simulink model "planning"  (R2018b)
settings: Solver=FixedStepDiscrete  StartTime=0.0  StopTime=10.0  RelTol=1e-3
settings Model: ExtModeTrigDuration=2  Creator=sin29  LastModifiedBy=sin29
settings OptimizationCC: DefaultParameterBehavior=Inlined  UseDivisionForNetSlopeComputation=on  UseFloatMulNetSlope=on  InlineInvariantSignals=on  PassReuseOutputArgsAs=Individual arguments  ZeroExternalMemoryAtStartup=off  ZeroInternalMemoryAtStartup=off  NoFixptDivByZeroProtection=on  EfficientFloat2IntCast=on  LifeSpan=1  MaxStackSize=64  OptimizeBlockOrder=speed  DifferentSizesBufferReuse=on
settings DebuggingCC: ParameterTunabilityLossMsg=error
settings HardwareCC: ProdBitPerInt=16  ProdBitPerPointer=16  ProdBitPerSizeT=16  ProdBitPerPtrDiffT=16  ProdLargestAtomicFloat=None  ProdWordSize=8  ProdLongLongMode=on  ProdHWDeviceType=Atmel->AVR
settings SFSimCC: MATLABDynamicMemAlloc=off
settings RTWCC: SystemTargetFile=ert.tlc  HardwareBoard=Arduino Uno  TemplateMakefile=ert_default_tmf  GenerateReport=on  Toolchain=Arduino AVR  BuildConfiguration=Faster Runs  IncludeHyperlinkInReport=on  LaunchReport=on  GenerateTraceInfo=on  GenerateTraceReport=on  GenerateTraceReportSl=on  GenerateTraceReportSf=on  GenerateTraceReportEml=on  GenerateCodeMetricsReport=on
settings CodeAppCC: ForceParamTrailComments=on  IgnoreCustomStorageClasses=off  OperatorAnnotations=on  SimulinkDataObjDesc=on  SFDataObjDesc=on  CustomSymbolStrGlobalVar=rt$N$M  CustomSymbolStrType=$N$M  CustomSymbolStrFcn=$N$M$F  CustomSymbolStrMacro=$N$M  InsertBlockDesc=on
settings ERTTargetCC: IncludeMdlTerminateFcn=off  CombineSignalStateStructs=on  SupportAbsoluteTime=off  SupportComplex=off  SupportNonInlinedSFcns=on  InlinedParameterPlacement=NonHierarchical  ERTFilePackagingFormat=CompactWithDataFile

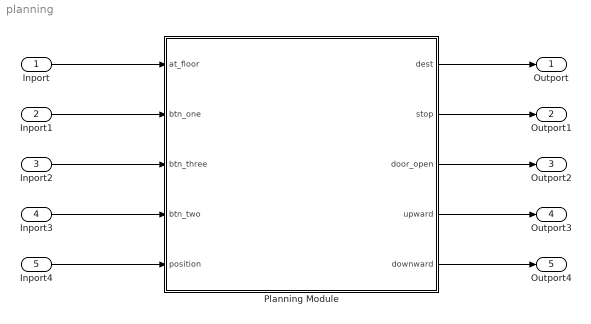
== system planning ==
  Inport : Inport
  Inport1 : Inport  Port=2
  Inport2 : Inport  Port=3
  Inport3 : Inport  Port=4
  Inport4 : Inport  Port=5
  "Planning Module " : Stateflow chart  TreatAsAtomicUnit=on
  Outport : Outport
  Outport1 : Outport  Port=2
  Outport2 : Outport  Port=3
  Outport3 : Outport  Port=4
  Outport4 : Outport  Port=5
  wires:
  Inport/1 -> "Planning Module "/1(at_floor)
  Inport1/1 -> "Planning Module "/2(btn_one)
  Inport2/1 -> "Planning Module "/3(btn_three)
  Inport3/1 -> "Planning Module "/4(btn_two)
  Inport4/1 -> "Planning Module "/5(position)
  "Planning Module "/1(dest) -> Outport/1
  "Planning Module "/2(stop) -> Outport1/1
  "Planning Module "/3(door_open) -> Outport2/1
  "Planning Module "/4(upward) -> Outport3/1
  "Planning Module "/5(downward) -> Outport4/1

== stateflow chart planning/Planning Module  ==
  state planning_cal
    state plan_handle [parallel]
      settings: executionOrder=1
      state floor1
        entry:
        one_pressed = 0;
        door_open = 1;
        stop = 1;
      state floor3
        entry:
        three_pressed = 0;
        door_open = 1;
        stop = 1;
      state move_up
        entry:
        door_open = 0;
        stop = 0;
        upward = 1;
        downward = 0;
      state move_down
        entry:
        door_open = 0;
        stop = 0;
        upward = 0;
        downward = 1;
      state floor2
        entry:
        two_pressed = 0;
        door_open = 1;
        stop = 1;
      floor1 -> floor1 [order 1] : [one_pressed == 1]
      (default) -> floor1
      floor1 -> move_up [order 2] : [after(5, sec) && two_pressed == 1]{dest = 2; two_open = 1}
      move_down -> floor1 [order 3] : [one_pressed == 1 && at_floor == 1]
      floor1 -> move_up [order 3] : [after(5, sec) && two_pressed == 0 && three_pressed == 1]{dest = 3; two_open = 0}
      floor3 -> floor3 [order 1] : [three_pressed == 1]
      move_up -> move_up [order 1] : [two_pressed == 1 && two_open == 0 && position <= 200]{two_open = 1; dest = 2}
      move_up -> floor3 [order 3] : [three_pressed == 1 && at_floor == 3]
      floor3 -> move_down [order 2] : [after(5, sec) && two_pressed == 0 && one_pressed == 1]{dest = 1; two_open = 0}
      floor3 -> move_down [order 3] : [after(5, sec) && two_pressed == 1]{dest = 2; two_open = 1}
      floor2 -> move_up [order 2] : [after(5, sec) && three_pressed == 1]{dest = 3}
      move_up -> floor2 [order 2] : [at_floor == 2 && two_pressed == 1 && two_open == 1]
      floor2 -> floor2 [order 1] : [two_pressed == 1]
      move_down -> floor2 [order 1] : [at_floor == 2 && two_pressed == 1 && two_open == 1]
      move_down -> move_down [order 2] : [two_pressed == 1 && two_open == 0 && position >= 600]{two_open = 1; dest = 2}
      floor2 -> move_down [order 3] : [after(5, sec) && one_pressed == 1]{dest = 1}
    state btn_handle [parallel]
      settings: executionOrder=2
      state btn_handle
      (default) -> planning_cal.btn_handle.btn_handle
      planning_cal.btn_handle.btn_handle -> planning_cal.btn_handle.btn_handle [order 1] : [btn_two == 1]{two_pressed = 1}
      planning_cal.btn_handle.btn_handle -> planning_cal.btn_handle.btn_handle [order 3] : [btn_one == 1]{one_pressed = 1}
      planning_cal.btn_handle.btn_handle -> planning_cal.btn_handle.btn_handle [order 2] : [btn_three == 1]{three_pressed = 1}
  state init
    exit:
    one_pressed = 0;
    two_pressed = 0;
    three_pressed = 0;
  (default) -> init
  init -> planning_cal
  data: at_floor input; btn_one input; btn_three input; btn_two input; position input; dest output; stop output; door_open output; upward output; downward output; two_pressed local; two_open local; three_pressed local; one_pressed local
